simulink model "Project_Part1"  (R2021a)
settings: Solver=VariableStepAuto  StartTime=0.0  StopTime=10.0  MaxStep=1e-3  RelTol=1e-3
settings Model: Creator=MAC  LastModifiedBy=MAC

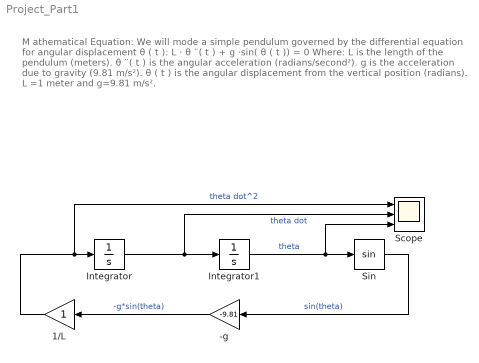
== system Project_Part1 ==
  note: M athematical Equation:
      | We will mode a simple pendulum governed by the differential equation for angular displacement θ ( t ):
      | L ⋅ θ ¨( t ) + g ⋅sin( θ ( t )) = 0
      | Where:
      | L is the length of the pendulum (meters).
      | θ ¨( t ) is the angular acceleration (radians/second²).
      | g is the acceleration due to gravity (9.81 m/s²).
      | θ ( t ) is the angular displacement from the vertical position (radians).
      | L =1 meter and g=9.81 m/s².
  -g : Gain  Gain=-9.81
  1/L : Gain
  Integrator : Integrator
  Integrator1 : Integrator  InitialCondition=40
  Scope : Scope  NumInputPorts=3
  Sin : Trigonometry
  wires:
  Integrator1/1 -> Scope/3, Sin/1  "theta"
  Integrator/1 -> Scope/2, Integrator1/1  "theta dot"
  1/L/1 -> Scope/1, Integrator/1  "theta dot^2"
  Sin/1 -> -g/1  "sin(theta)"
  -g/1 -> 1/L/1  "-g*sin(theta)"
